simulink model "System"  (R2025b)
settings: Solver=ode8  StartTime=0.0  StopTime=2*60  FixedStep=1  RelTol=1e-3
model workspace (MAT data in the model file):
  Sig = Simulink.Signal
  Sig.Dimensions = -1
  Sig.DimensionsMode = 'auto'
  Sig.Complexity = 'auto'
  Sig.SampleTime = -1
  Sig.SamplingMode = 'auto'
  Sig.DataType = 'auto'
settings Model: Creator=Soere  LastModifiedBy=klump
settings DebuggingCC: UnderSpecifiedDimensionMsg=warning

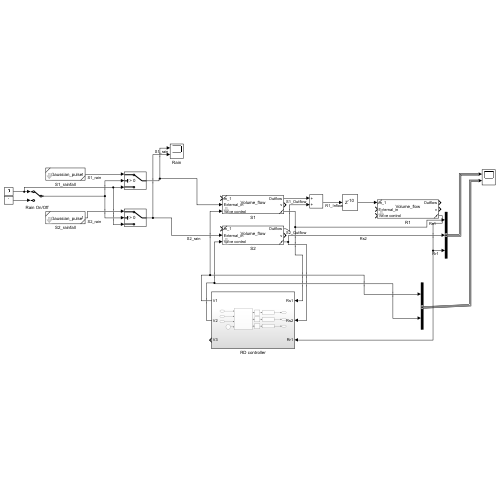
[thumbnail: Simulink's stored preview of the top-level diagram]
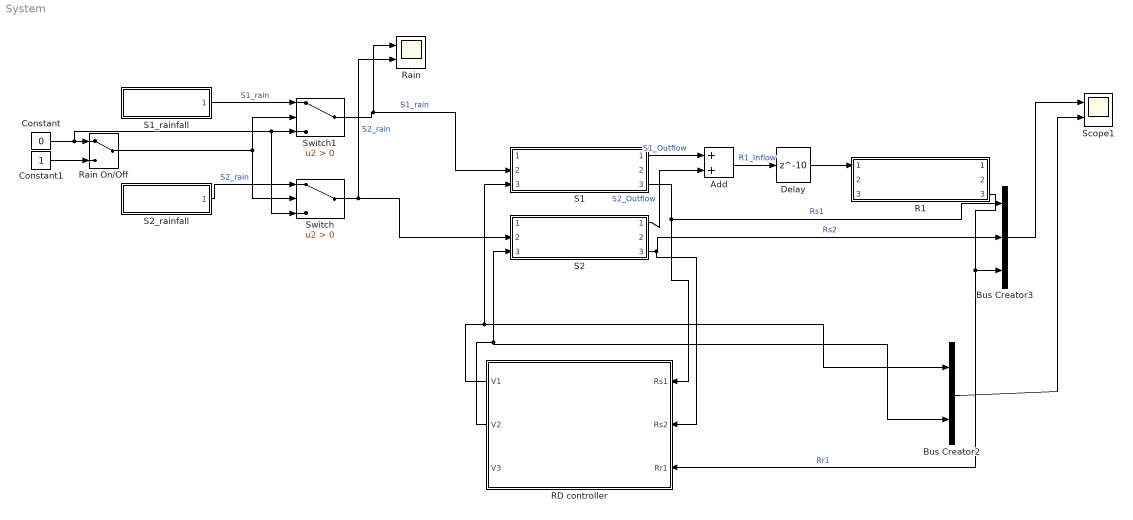
== system System ==
  Add : Sum
  Bus Creator2 : BusCreator  Inputs=2
  Bus Creator3 : BusCreator  Inputs=3
  Constant : Constant  Value=0
  Constant1 : Constant
  Delay : Delay  DelayLength=10  InputProcessing=Columns as channels (frame based)
  R1 : Subsystem  ReferencedSubsystem=Volume_flow  InitialCondition=0  Gain_k=0.005  Gain_y=0  Max_cap=300
  RD controller : Subsystem
  Rain : Scope  NumInputPorts=2
      settings: ActiveDisplayYMinimum=-1  ActiveDisplayYMaximum=1  DataLoggingVariableName=ScopeData8
  Rain On/Off : ManualSwitch
  S1 : Subsystem  ReferencedSubsystem=Volume_flow  InitialCondition=275  Gain_k=0.009  Gain_y=0  Max_cap=300
  S1_rainfall : Subsystem  ReferencedSubsystem=Gaussian_pulse  PeakTime=0.5*60  Amplitude=5  Sigma=60*0.3
  S2 : Subsystem  ReferencedSubsystem=Volume_flow  InitialCondition=150  Gain_k=0.009  Gain_y=0  Max_cap=300
  S2_rainfall : Subsystem  ReferencedSubsystem=Gaussian_pulse  PeakTime=0.3*60  Amplitude=4  Sigma=60*0.3
  Scope1 : Scope  NumInputPorts=2
      settings: ActiveDisplayYMaximum=310  DataLoggingVariableName=ScopeData7
  Switch : Switch  Criteria=u2 > Threshold  SaturateOnIntegerOverflow=off  InputSameDT=off
  Switch1 : Switch  Criteria=u2 > Threshold  SaturateOnIntegerOverflow=off  InputSameDT=off
  wires:
  S1/1 -> Add/1  "S1_Outflow"
  S2/1 -> Add/2  "S2_Outflow"
  Add/1 -> Delay/1  "R1_Inflow"
  Bus Creator2/1 -> Scope1/2
  Switch1/1 -> S1/2, Rain/1  "S1_rain"
  Switch/1 -> S2/2, Rain/2  "S2_rain"
  S1_rainfall/1 -> Switch1/1  "S1_rain"
  S2_rainfall/1 -> Switch/1  "S2_rain"
  Bus Creator3/1 -> Scope1/1
  R1/3 -> RD controller/3(Rr1), Bus Creator3/3  "Rr1"
  S2/3 -> RD controller/2(Rs2), Bus Creator3/2  "Rs2"
  S1/3 -> RD controller/1(Rs1), Bus Creator3/1  "Rs1"
  Rain On/Off/1 -> Switch/2, Switch1/2
  Constant/1 -> Switch/3, Switch1/3, Rain On/Off/1
  Constant1/1 -> Rain On/Off/2
  RD controller/1(V1) -> Bus Creator2/1, S1/3
  RD controller/2(V2) -> S2/3, Bus Creator2/2
  Delay/1 -> R1/1

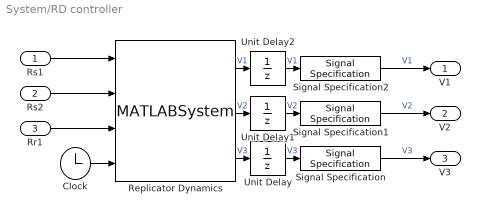
== system System/RD controller ==
  Rs1 : Inport
  Rs2 : Inport  Port=2
  Rr1 : Inport  Port=3
  Clock : Clock
  Replicator Dynamics : MATLABSystem  System=controller  SimulateUsing=Interpreted execution
      mask Type: controller
  Signal Specification : SignalSpecification  Dimensions=1
  Signal Specification1 : SignalSpecification  Dimensions=1
  Signal Specification2 : SignalSpecification  Dimensions=1
  Unit Delay : UnitDelay  SampleTime=-1  HasFrameUpgradeWarning=on
  Unit Delay1 : UnitDelay  SampleTime=-1  HasFrameUpgradeWarning=on
  Unit Delay2 : UnitDelay  SampleTime=-1  HasFrameUpgradeWarning=on
  V1 : Outport
  V2 : Outport  Port=2
  V3 : Outport  Port=3
  wires:
  Unit Delay/1 -> Signal Specification/1  "V3"
  Unit Delay2/1 -> Signal Specification2/1  "V1"
  Clock/1 -> Replicator Dynamics/4
  Rs1/1 -> Replicator Dynamics/1
  Replicator Dynamics/1 -> Unit Delay2/1  "V1"
  Unit Delay1/1 -> Signal Specification1/1  "V2"
  Replicator Dynamics/2 -> Unit Delay1/1  "V2"
  Replicator Dynamics/3 -> Unit Delay/1  "V3"
  Rs2/1 -> Replicator Dynamics/2
  Rr1/1 -> Replicator Dynamics/3
  Signal Specification2/1 -> V1/1  "V1"
  Signal Specification/1 -> V3/1  "V3"
  Signal Specification1/1 -> V2/1  "V2"
